simulink model "homework5model"  (R2018a)
settings: Solver=VariableStepAuto  StartTime=0.0  StopTime=30  RelTol=1e-3
undefined symbols (not defined in the file or in its folder): denG, denGfb, denGff, numG, numGfb, numGff
settings Model: Creator=milos  LastModifiedBy=milos

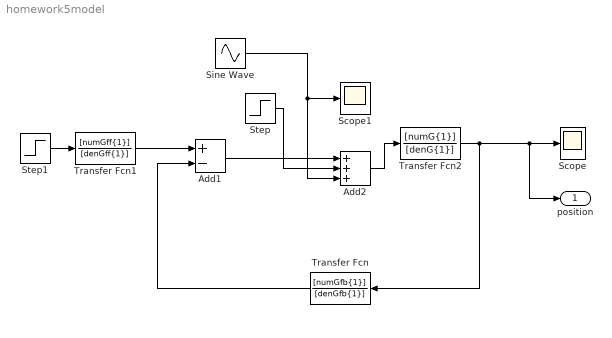
== system homework5model ==
  Add1 : Sum  Inputs=+-
  Add2 : Sum  Inputs=+++
  Scope : Scope
  Scope1 : Scope
  Sine Wave : Sin  SampleTime=0
  Step : Step  Time=0  SampleTime=0
  Step1 : Step  Time=0  SampleTime=0
  Transfer Fcn : TransferFcn  Numerator=[numGfb{1}]  Denominator=[denGfb{1}]
  Transfer Fcn1 : TransferFcn  Numerator=[numGff{1}]  Denominator=[denGff{1}]
  Transfer Fcn2 : TransferFcn  Numerator=[numG{1}]  Denominator=[denG{1}]
  position : Outport
  wires:
  Add1/1 -> Add2/1
  Sine Wave/1 -> Add2/3, Scope1/1
  Transfer Fcn/1 -> Add1/2
  Transfer Fcn1/1 -> Add1/1
  Step1/1 -> Transfer Fcn1/1
  Step/1 -> Add2/2
  Add2/1 -> Transfer Fcn2/1
  Transfer Fcn2/1 -> Transfer Fcn/1, position/1, Scope/1
